simulink model "QuadrotorOwnDynamicModel"  (Simulink 9.0)
settings: Solver=ode45  StartTime=0.0  StopTime=5.0  RelTol=1e-3  EnableMultiTasking=on
values from neighbouring files (symbols this model uses):
  b = 1.14e-07    [ParLuk11.m]
  Ixx = 4.856e-03    (= 0.004856)    [ParLuk11.m]
  Iyy = Ixx    (= 0.004856)    [ParLuk11.m]
  Izz = 8.801e-03    (= 0.008801)    [ParLuk11.m]
  k = 2.98e-06    [ParLuk11.m]
  L = 0.225    [ParLuk11.m]
  m = 0.468    [ParLuk11.m]
libraries: vrlib x4
settings Model: Creator=Jan  LastModifiedBy=Jan
settings DataIOCC: LimitDataPoints=on
settings DebuggingCC: UnderspecifiedInitializationDetection=Simplified  MergeDetectMultiDrivingBlocksExec=error
settings GRTTargetCC: GeneratePreprocessorConditionals=Disable all

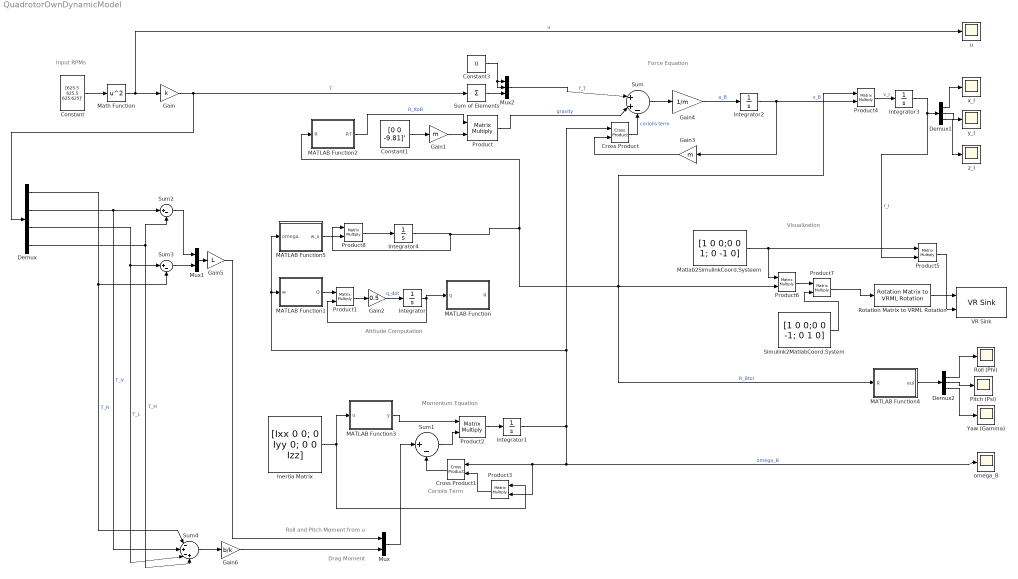
== system QuadrotorOwnDynamicModel ==
  note: Input RPMs
  note: Visualization
  note: Roll and Pitch Moment from u
  note: Drag Moment
  note: Coriolis Term
  note: Attitude Computation
  note: Momentum Equation
  note: Force Equation
  Constant : Constant  Value=[625.5 625.5 625 625]'  VectorParams1D=off
  Constant1 : Constant  Value=[0 0 -9.81]'  VectorParams1D=off
  Constant3 : Constant  Value=0
  Cross Product : vrlib/Utilities/Cross Product
      settings: SourceProductBaseCode=VR
  Cross Product1 : vrlib/Utilities/Cross Product
      settings: SourceProductBaseCode=VR
  Demux : Demux
  Demux1 : Demux  Outputs=3
  Demux2 : Demux  Outputs=3
  Gain : Gain  Gain=k
  Gain1 : Gain  Gain=m
  Gain2 : Gain  Gain=0.5
  Gain3 : Gain  Gain=m
  Gain4 : Gain  Gain=1/m
  Gain5 : Gain  Gain=L
  Gain6 : Gain  Gain=b/k
  Inertia Matrix : Constant  Value=[Ixx 0 0; 0 Iyy 0; 0 0 Izz]
  Integrator : Integrator  InitialCondition=[0 0 0 1]
  Integrator1 : Integrator  InitialCondition=[0 0 0]
  Integrator2 : Integrator
  Integrator3 : Integrator  InitialCondition=[0 0 0]'
  Integrator4 : Integrator  InitialCondition=[1 0 0; 0 1 0; 0 0 1]
  MATLAB Function : MATLAB Function  TreatAsAtomicUnit=on
  MATLAB Function1 : MATLAB Function  TreatAsAtomicUnit=on
  MATLAB Function2 : MATLAB Function  TreatAsAtomicUnit=on
  MATLAB Function3 : MATLAB Function  TreatAsAtomicUnit=on
  MATLAB Function4 : MATLAB Function  TreatAsAtomicUnit=on
  MATLAB Function5 : MATLAB Function  TreatAsAtomicUnit=on
  Math Function : Math  Operator=square  SaturateOnIntegerOverflow=on
  "Matlab2SimulinkCoord.Systeem " : Constant  Value=[1 0 0;0 0 1; 0 -1 0]  VectorParams1D=off
  Mux : Mux  Inputs=2
  Mux1 : Mux  Inputs=2
  Mux2 : Mux  Inputs=3
  Pitch (Psi) : Scope
  Product{,1..8} (9 alike) : Product  Multiplication=Matrix(*)
  Roll (Phi) : Scope
  Rotation Matrix to VRML Rotation : vrlib/Utilities/Rotation Matrix to VRML Rotation  maxzero=1e-12
      settings: SourceProductName=Simulink 3D Animation  SourceProductBaseCode=VR
  "Simulink2MatlabCoord.System " : Constant  Value=[1 0 0;0 0 -1; 0 1 0]  VectorParams1D=off
  Sum : Sum  Inputs=|++-
  Sum of Elements : Sum  Inputs=+
  Sum1 : Sum  Inputs=|+-
  Sum2 : Sum  Inputs=|+-
  Sum3 : Sum  Inputs=|+-
  Sum4 : Sum  Inputs=|-+-+
  VR Sink : vrlib/VR Sink  InstantiateOnLoad=on  SampleTime=0.1  ViewEnable=on  RemoteChange=off  RemoteView=off  FieldsWritten=Quadro.rotation.4.1.1.double#Quadro.translation.3.1.1.double  WorldFileName=vrmodell_first  AutoView=off  VideoDimensions=[]  AllowVariableSize=off  FigureProperties="{'Position', 'Name', 'Viewpoint', 'CameraBound', 'CameraDirection', 'CameraPosition', 'CameraUpVector', 'ZoomFactor', 'Antialiasing', 'Headlight', 'Lighting', 'NavPanel', 'Sound', 'StatusBar', 'Stereo3D', 'Stereo3DCameraOffset', 'Stereo3DHIT', 'ToolBar', 'Textures', 'Transparency', 'Triad', 'Wireframe', 'NavZones', 'NavMode', 'NavSpeed', 'CaptureFileFormat', 'CaptureFileName', 'Record2DCompressMethod', 'Record2DCompressQuality', 'Record2D', 'Record2DFileName', 'Record2DFPS'; [1.3290000000000000e+03   1.3700000000000000e+02   7.6100000000000000e+02   6.6100000000000000e+02], '', '_untitled_1', 'on', [0.0000000000000000e+00   0.0000000000000000e+00  -1.0000000000000000e+00], [0.0000000000000000e+00   0.0000000000000000e+00   0.0000000000000000e+00], [0.0000000000000000e+00   1.0000000000000000e+00   0.0000000000000000e+00], [1.0000000000000000e+00], 'on', 'on', 'on', 'halfbar', 'on', 'on', 'off', [1.0000000149011612e-01], [0.0000000000000000e+00], 'on', 'on', 'on', 'none', 'off', 'off', 'fly', 'normal', 'tif', '%f_anim_%n.tif', 'auto', [7.5000000000000000e+01], 'off', '%f_anim_%n.avi', 'auto'}"
      settings: SourceProductBaseCode=VR
  Yaw (Gamma) : Scope
  omega_B : Scope
  u : Scope
  x_I : Scope
  y_I : Scope
  z_I : Scope
  wires:
  Gain/1 -> Demux/1, Sum of Elements/1  "T"
  Constant1/1 -> Gain1/1
  Integrator4/1 -> Product4/1, Product6/2, MATLAB Function4/1(R), MATLAB Function2/1(R), Product8/1  "R_BtoI"
  Gain1/1 -> Product/2
  MATLAB Function2/1(RT) -> Product/1  "R_ItoB"
  Product/1 -> Sum/2  "gravity"
  Integrator/1 -> Product1/2, MATLAB Function/1(q)
  MATLAB Function1/1(Q) -> Product1/1
  Product1/1 -> Gain2/1
  Gain2/1 -> Integrator/1  "q_dot"
  Integrator1/1 -> omega_B/1, Product3/2, Cross Product1/1, MATLAB Function5/1(omega), MATLAB Function1/1(w), Cross Product/1  "omega_B"
  Gain3/1 -> Cross Product/2
  Integrator2/1 -> Product4/2, Gain3/1  "v_B"
  Cross Product/1 -> Sum/3  "coriolis term"
  Sum/1 -> Gain4/1
  Gain4/1 -> Integrator2/1  "a_B"
  Inertia Matrix/1 -> MATLAB Function3/1(u), Product3/1
  MATLAB Function3/1(y) -> Product2/1
  Sum1/1 -> Product2/2
  Product2/1 -> Integrator1/1
  Cross Product1/1 -> Sum1/2
  Product3/1 -> Cross Product1/2
  Mux/1 -> Sum1/1
  Gain5/1 -> Mux/1
  Mux1/1 -> Gain5/1
  Sum2/1 -> Mux1/1
  Demux/2 -> Sum2/1, Sum4/2  "T_V"
  Demux/4 -> Sum2/2, Sum4/4  "T_H"
  Sum3/1 -> Mux1/2
  Demux/3 -> Sum3/1, Sum4/3  "T_L"
  Demux/1 -> Sum4/1, Sum3/2  "T_R"
  Gain6/1 -> Mux/2
  Sum4/1 -> Gain6/1
  Constant/1 -> Math Function/1
  Math Function/1 -> Gain/1, u/1  "u"
  Integrator3/1 -> Product5/2, Demux1/1  "r_I"
  Demux1/1 -> x_I/1
  Demux1/2 -> y_I/1
  Demux1/3 -> z_I/1
  Constant3/1 -> Mux2/2, Mux2/1
  Sum of Elements/1 -> Mux2/3
  Mux2/1 -> Sum/1  "f_T"
  Product5/1 -> VR Sink/2
  Rotation Matrix to VRML Rotation/1 -> VR Sink/1
  Product4/1 -> Integrator3/1  "v_I"
  MATLAB Function4/1(eul) -> Demux2/1
  Demux2/1 -> Roll (Phi)/1
  Demux2/2 -> Pitch (Psi)/1
  Demux2/3 -> Yaw (Gamma)/1
  "Matlab2SimulinkCoord.Systeem "/1 -> Product5/1, Product6/1
  Product6/1 -> Product7/1
  Product7/1 -> Rotation Matrix to VRML Rotation/1
  "Simulink2MatlabCoord.System "/1 -> Product7/2
  MATLAB Function5/1(w_x) -> Product8/2
  Product8/1 -> Integrator4/1

== matlab function MATLAB Function1 ==
  data: w input double; Q output double
function Q = omegaSkew(w)
%#codegen

Q = [0 w(3) -w(2) w(1);
    -w(3) 0 w(1) w(2);
    w(2) -w(1) 0 w(3);
    -w(1) -w(2) -w(3) 0];

== matlab function MATLAB Function ==
  data: q input double; R output double
function R = Quat2R(q)
% compute R from quaternion input

R = [q(1)^2 - q(2)^2 - q(3)^2 + q(4)^2,  2*(q(1)*q(2) - q(3)*q(4)),          2*(q(1)*q(3) + q(2)*q(4));
     2*(q(1)*q(2) + q(3)*q(4)),         -q(1)^2 + q(2)^2 - q(3)^2 + q(4)^2,  2*(q(2)*q(3) - q(1)*q(4));
     2*(q(1)*q(3) - q(2)*q(4)),          2*(q(2)*q(3) + q(1)*q(4)),         -q(1)^2 - q(2)^2 + q(3)^2 + q(4)^2];

== matlab function MATLAB Function2 ==
  data: R input double; RT output double
function RT = transpose(R)
%#codegen

RT = R';

== matlab function MATLAB Function3 ==
  data: u input double; y output double
function y = inverse(u)
%#codegen

y = inv(u);

== matlab function MATLAB Function4 ==
  data: R input double; eul output double
function eul = DCM2Euler(R)

%Roll
phi = atan2d(R(3,2),R(3,3));

%Pitch
psi = atan2d(-R(3,1),sqrt(R(1,1)^2 + R(2,1)^2));

%Yaw
gamma = atan2d(R(2,1),R(1,1));

eul=[phi;psi;gamma];

== matlab function MATLAB Function5 ==
  data: omega input double; w_x output double
function w_x = omegaSkew3D(omega)

w_x = [0 -omega(3) omega(2);
        omega(3) 0 -omega(1);
        -omega(2) omega(1) 0];
